simulink library "lib_util"  (Simulink 7.7)
settings: Solver=ode45  StartTime=0.0  StopTime=10.0  RelTol=1e-3
libraries: lib_util x6, aerolibutil x1
settings Model: Creator=kkamiya  LastModifiedBy=yamaurashusaku

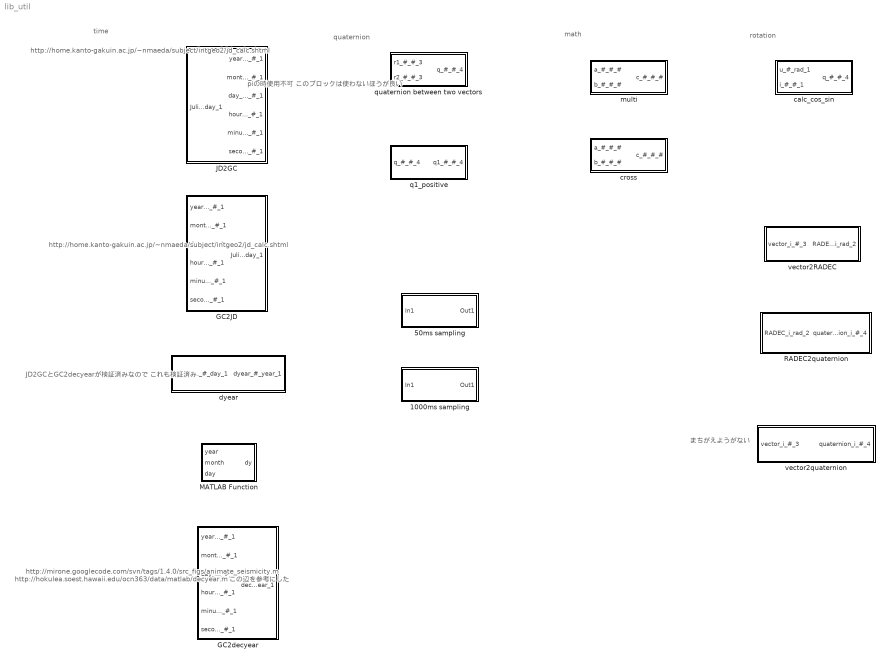
== system lib_util ==
  note: time
  note: quaternion
  note: math
  note: rotation
  note: http://home.kanto-gakuin.ac.jp/~nmaeda/subject/intgeo2/jd_calc.shtml
  note: http://home.kanto-gakuin.ac.jp/~nmaeda/subject/intgeo2/jd_calc.shtml
  note: http://mirone.googlecode.com/svn/tags/1.4.0/src_figs/animate_seismicity.m
      | http://hokulea.soest.hawaii.edu/ocn363/data/matlab/decyear.m
      | この辺を参考にした
  note: JD2GCとGC2decyearが検証済みなので
      | これも検証済み
  note: piの時使用不可
      | このブロックは使わないほうが良い
  note: まちがえようがない
  1000ms sampling : Subsystem
  50ms sampling : Subsystem
  GC2JD : Subsystem
  GC2decyear : Subsystem
  JD2GC : Subsystem
  MATLAB Function : Stateflow chart  TreatAsAtomicUnit=on
  RADEC2quaternion : Subsystem
  calc_cos_sin : Subsystem
  cross : Subsystem
  dyear : Subsystem
  multi : Subsystem
  q1_positive : Subsystem
  quaternion between two vectors : Subsystem
  vector2RADEC : Subsystem
  vector2quaternion : Subsystem

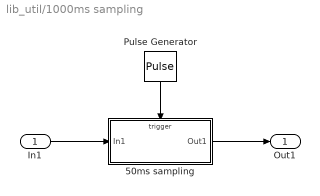
== system lib_util/1000ms sampling ==
  In1 : Inport
  50ms sampling : Subsystem  TreatAsAtomicUnit=on
  Pulse Generator : DiscretePulseGenerator  PulseType=Time based  Period=1  PulseWidth=20
  Out1 : Outport
  wires:
  50ms sampling/1(Out1) -> Out1/1
  In1/1 -> 50ms sampling/1(In1)
  Pulse Generator/1 -> 50ms sampling/Trigger

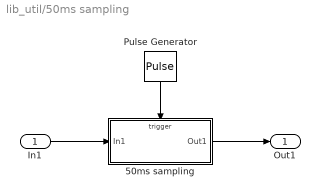
== system lib_util/50ms sampling ==
  In1 : Inport
  50ms sampling : Subsystem  TreatAsAtomicUnit=on
  Pulse Generator : DiscretePulseGenerator  PulseType=Time based  Period=0.05  PulseWidth=20
  Out1 : Outport
  wires:
  Pulse Generator/1 -> 50ms sampling/Trigger
  In1/1 -> 50ms sampling/1(In1)
  50ms sampling/1(Out1) -> Out1/1

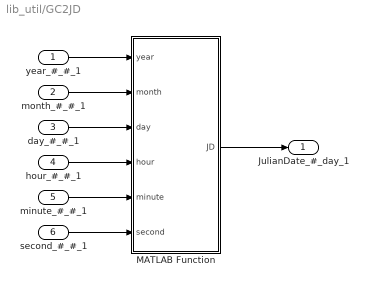
== system lib_util/GC2JD ==
  year_#_#_1 : Inport
  month_#_#_1 : Inport  Port=2
  day_#_#_1 : Inport  Port=3
  hour_#_#_1 : Inport  Port=4
  minute_#_#_1 : Inport  Port=5
  second_#_#_1 : Inport  Port=6
  MATLAB Function : Stateflow chart  TreatAsAtomicUnit=on
  JulianDate_#_day_1 : Outport
  wires:
  MATLAB Function/1(JD) -> JulianDate_#_day_1/1
  second_#_#_1/1 -> MATLAB Function/6(second)
  minute_#_#_1/1 -> MATLAB Function/5(minute)
  hour_#_#_1/1 -> MATLAB Function/4(hour)
  day_#_#_1/1 -> MATLAB Function/3(day)
  month_#_#_1/1 -> MATLAB Function/2(month)
  year_#_#_1/1 -> MATLAB Function/1(year)

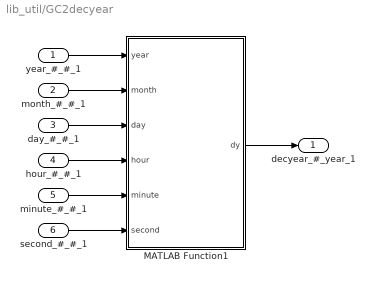
== system lib_util/GC2decyear ==
  year_#_#_1 : Inport
  month_#_#_1 : Inport  Port=2
  day_#_#_1 : Inport  Port=3
  hour_#_#_1 : Inport  Port=4
  minute_#_#_1 : Inport  Port=5
  second_#_#_1 : Inport  Port=6
  MATLAB Function1 : Stateflow chart  TreatAsAtomicUnit=on
  decyear_#_year_1 : Outport
  wires:
  MATLAB Function1/1(dy) -> decyear_#_year_1/1
  second_#_#_1/1 -> MATLAB Function1/6(second)
  minute_#_#_1/1 -> MATLAB Function1/5(minute)
  hour_#_#_1/1 -> MATLAB Function1/4(hour)
  day_#_#_1/1 -> MATLAB Function1/3(day)
  month_#_#_1/1 -> MATLAB Function1/2(month)
  year_#_#_1/1 -> MATLAB Function1/1(year)

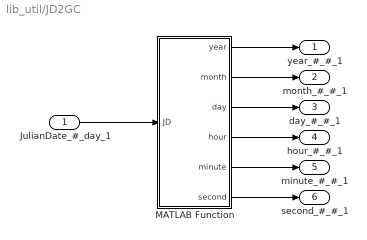
== system lib_util/JD2GC ==
  JulianDate_#_day_1 : Inport
  MATLAB Function : Stateflow chart  TreatAsAtomicUnit=on
  year_#_#_1 : Outport
  month_#_#_1 : Outport  Port=2
  day_#_#_1 : Outport  Port=3
  hour_#_#_1 : Outport  Port=4
  minute_#_#_1 : Outport  Port=5
  second_#_#_1 : Outport  Port=6
  wires:
  JulianDate_#_day_1/1 -> MATLAB Function/1(JD)
  MATLAB Function/6(second) -> second_#_#_1/1
  MATLAB Function/5(minute) -> minute_#_#_1/1
  MATLAB Function/4(hour) -> hour_#_#_1/1
  MATLAB Function/3(day) -> day_#_#_1/1
  MATLAB Function/2(month) -> month_#_#_1/1
  MATLAB Function/1(year) -> year_#_#_1/1

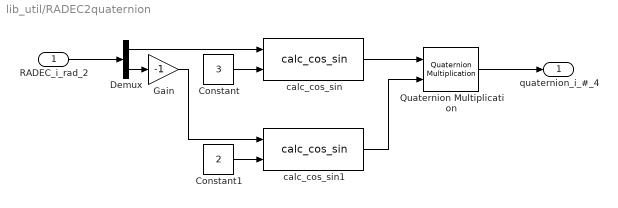
== system lib_util/RADEC2quaternion ==
  RADEC_i_rad_2 : Inport
  Constant : Constant  Value=3
  Constant1 : Constant  Value=2
  Demux : Demux  Outputs=2
  Gain : Gain  Gain=-1
  Quaternion Multiplication : aerolibutil/Quaternion Multiplication
  calc_cos_sin : lib_util/calc_cos_sin
  calc_cos_sin1 : lib_util/calc_cos_sin
  quaternion_i_#_4 : Outport
  wires:
  RADEC_i_rad_2/1 -> Demux/1
  Demux/1 -> calc_cos_sin/1
  Constant/1 -> calc_cos_sin/2
  Demux/2 -> Gain/1
  Constant1/1 -> calc_cos_sin1/2
  Quaternion Multiplication/1 -> quaternion_i_#_4/1
  calc_cos_sin/1 -> Quaternion Multiplication/1
  calc_cos_sin1/1 -> Quaternion Multiplication/2
  Gain/1 -> calc_cos_sin1/1

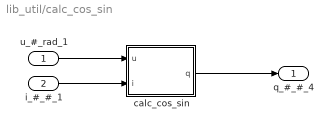
== system lib_util/calc_cos_sin ==
  u_#_rad_1 : Inport
  i_#_#_1 : Inport  Port=2
  calc_cos_sin : Stateflow chart  TreatAsAtomicUnit=on
  q_#_#_4 : Outport
  wires:
  u_#_rad_1/1 -> calc_cos_sin/1(u)
  calc_cos_sin/1(q) -> q_#_#_4/1
  i_#_#_1/1 -> calc_cos_sin/2(i)

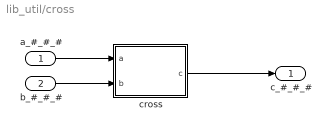
== system lib_util/cross ==
  a_#_#_# : Inport
  b_#_#_# : Inport  Port=2
  cross : Stateflow chart  TreatAsAtomicUnit=on
  c_#_#_# : Outport
  wires:
  a_#_#_#/1 -> cross/1(a)
  b_#_#_#/1 -> cross/2(b)
  cross/1(c) -> c_#_#_#/1

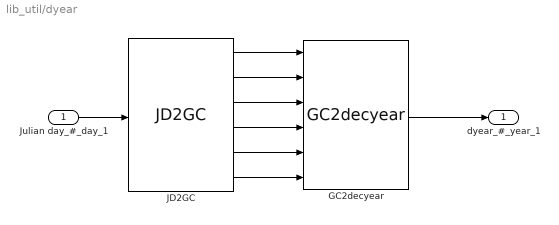
== system lib_util/dyear ==
  Julian day_#_day_1 : Inport
  GC2decyear : lib_util/GC2decyear
  JD2GC : lib_util/JD2GC
  dyear_#_year_1 : Outport
  wires:
  Julian day_#_day_1/1 -> JD2GC/1
  JD2GC/1 -> GC2decyear/1
  JD2GC/2 -> GC2decyear/2
  JD2GC/3 -> GC2decyear/3
  JD2GC/4 -> GC2decyear/4
  JD2GC/5 -> GC2decyear/5
  JD2GC/6 -> GC2decyear/6
  GC2decyear/1 -> dyear_#_year_1/1

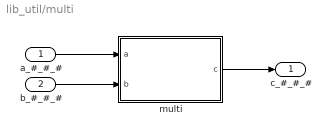
== system lib_util/multi ==
  a_#_#_# : Inport
  b_#_#_# : Inport  Port=2
  multi : Stateflow chart  TreatAsAtomicUnit=on
  c_#_#_# : Outport
  wires:
  b_#_#_#/1 -> multi/2(b)
  a_#_#_#/1 -> multi/1(a)
  multi/1(c) -> c_#_#_#/1

== system lib_util/q1_positive ==
  q_#_#_4 : Inport
  q1_positive : Stateflow chart  TreatAsAtomicUnit=on
  q1_#_#_4 : Outport
  wires:
  q_#_#_4/1 -> q1_positive/1(q)
  q1_positive/1(q1) -> q1_#_#_4/1

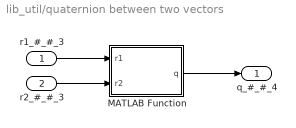
== system lib_util/quaternion between two vectors ==
  r1_#_#_3 : Inport
  r2_#_#_3 : Inport  Port=2
  MATLAB Function : Stateflow chart  TreatAsAtomicUnit=on
  q_#_#_4 : Outport
  wires:
  MATLAB Function/1(q) -> q_#_#_4/1
  r2_#_#_3/1 -> MATLAB Function/2(r2)
  r1_#_#_3/1 -> MATLAB Function/1(r1)

== system lib_util/vector2RADEC ==
  vector_i_#_3 : Inport
  MATLAB Function : Stateflow chart  TreatAsAtomicUnit=on
  RADEC_i_rad_2 : Outport
  wires:
  vector_i_#_3/1 -> MATLAB Function/1(r)
  MATLAB Function/1(RADEC) -> RADEC_i_rad_2/1

== system lib_util/vector2quaternion ==
  vector_i_#_3 : Inport
  RADEC2quaternion : lib_util/RADEC2quaternion
  vector2RADEC : lib_util/vector2RADEC
  quaternion_i_#_4 : Outport
  wires:
  vector_i_#_3/1 -> vector2RADEC/1
  vector2RADEC/1 -> RADEC2quaternion/1
  RADEC2quaternion/1 -> quaternion_i_#_4/1

== system lib_util/1000ms sampling/50ms sampling ==
  In1 : Inport
  Trigger : TriggerPort
  Out1 : Outport
  wires:
  In1/1 -> Out1/1

== system lib_util/50ms sampling/50ms sampling ==
  In1 : Inport
  Trigger : TriggerPort
  Out1 : Outport
  wires:
  In1/1 -> Out1/1

== matlab function quaternion between two vectors/MATLAB Function ==
  data: r1 input double; q output double; r2 input double
function q = fcn(r1, r2)
%#codegen

cosphi = dot(r1, r2);
if cosphi > 1.0
    cosphi = 1.0;
end
if cosphi < -1.0
    cosphi = -1.0;
end

phi = acos(cosphi);

r3 = cross(r1, r2);

if cosphi < -1.0 + 1.0e-2
    max = -1.0e+10;
    min = 1.0e+10;
    maxi = -1;
    midi = -1;
    mini = -1;
    
    for i=1:3
        fabs = abs(r1(i));
        if max < fabs
            max = fabs;
            maxi = i;
        end
        if min > fabs
            min = fabs;
            mini = i;
        end
    end
    
    for i=1:3
        if i ~= maxi
            if i ~= mini
                midi = i;
            end
        end
    end
    
    r3(mini) = 0.0;
    r3(midi) = sqrt(r1(maxi) * r1(maxi) / (r1(maxi) * r1(maxi) + r1(midi) * r1(midi)));
    r3(maxi) = -r1(midi) / r1(maxi) * r3(midi);
    
end

cph = cos(phi / 2.0);
sph = sin(phi / 2.0);
q = [cph, r3(1) * sph, r3(2) * sph, r3(3) * sph];

== matlab function JD2GC/MATLAB Function ==
  data: JD input double; year output double; month output double; day output double; hour output double; minute output double; second output double
function [year,month,day,hour,minute,second]= JD2GC(JD)
%#codegen

fday   = JD + 0.5 - floor(JD + 0.5) ;
JD     = floor(JD + 0.5);
in2    = floor(floor((JD - 4479.5) / 36524.25) * 0.75 + 0.5) - 37;
in2    = JD + in2;
year   = floor(in2 / 365.25) - 4712;
an2    = in2 - 59.25;
an2    = floor(an2 - floor(an2 / 365.25) * 365.25) + 0.5;
mon2   = floor(an2 / 30.6) + 2;
month  = mon2 - floor(mon2 / 12) * 12 + 1;
day    = floor(an2 - floor(an2 / 30.6) * 30.6 + 1);
hour   = floor(fday * 24);
minute = floor((fday * 24 - floor(fday * 24)) * 60) ;
second = fday * 24 * 60 * 60 - floor(fday * 24) * 60 * 60 ...
    - floor((fday * 24 - floor(fday * 24)) * 60) * 60;

== matlab function GC2JD/MATLAB Function ==
  data: year input double; JD output double; month input double; day input double; hour input double; minute input double; second input double
function JD = GC2JD(year, month, day, hour, minute, second)
%#codegen

mm  = fix((month - 14) / 12);
MJD = fix(1461 * (year + 4800 + mm) / 4);
MJD = MJD + fix(367 * (month - 2 - mm * 12) / 12);
MJD = MJD - fix(3 * fix((year + 4900 + mm) / 100) / 4) - 2432076 + day;

JD = MJD + 2400000.5 + (hour + minute / 60 + second / 3600.0) / 24;

== matlab function MATLAB Function ==
  data: year input double; dy output double; month input double; day input double
function dy = DOY(year, month, day)
%#codegen

days_in_prev_months = [0 31 59 90 120 151 181 212 243 273 304 334]';

% Day in given month.
dy = days_in_prev_months(month) ...                % days in prev. months
   + (isleapyear(year) & (month > 2)) ...          % leap day
   + day;                                          % day in month

function t = isleapyear(year)
	t = (~rem(year, 4) & rem(year, 100)) | ~rem(year, 400);

== matlab function multi/multi ==
  data: a input double; c output double; b input double
function c  = multi(a,b)
%#codegen
c=a*b;

== matlab function vector2RADEC/MATLAB Function ==
  data: r input double; RADEC output double
function RADEC = vector2RADEC(r)
%#codegen

RA  = atan2(r(2), r(1));
DEC = asin(r(3) / sqrt(r(1)^2 + r(2)^2 + r(3)^2));

RADEC = [RA; DEC];

== matlab function GC2decyear/MATLAB Function1 ==
  data: dy output double; year input double; month input double; day input double; hour input double; minute input double; second input double
function dy = dec_year(year, month, day, hour, minute, second)
%#codegen

days_in_prev_months = [0 31 59 90 120 151 181 212 243 273 304 334]';

% Day in given month.
dy = days_in_prev_months(month) ...                % days in prev. months
   + (isleapyear(year) & (month > 2)) ...          % leap day
   + day ...                                       % day in month
   + (second + 60 * minute + 3600 * hour) / 86400; % part of day
dy = year + (dy - 1) / (365 + isleapyear(year));

function t = isleapyear(year)
	t = (~rem(year, 4) & rem(year, 100)) | ~rem(year, 400);

== matlab function q1_positive/q1_positive ==
  data: q input double; q1 output double
function q1 = fcn(q)
%#codegen

if q(1) <0
    q1=-q;
else
    q1=q;
end

== matlab function calc_cos_sin/calc_cos_sin ==
  data: u input double; q output double; i input double
function q = sankaku(u,i)
%#codegen
u=u/2;
if i == 1
   q=[cos(u);sin(u);0;0]; 
elseif i == 2
   q=[cos(u);0;sin(u);0];
else
   q=[cos(u);0;0;sin(u)];    
end

== matlab function cross/cross ==
  data: a input double; b input double; c output double
function c = fcn(a,b)
%#codegen

c =cross(a,b);
